simulink model "Simulink_Serial_Example"  (R2018b)
settings: Solver=VariableStepAuto  StartTime=0.0  StopTime=inf  RelTol=1e-3
undefined symbols (not defined in the file or in its folder): serial
libraries: instrumentlib x3
settings Model: Creator=root  LastModifiedBy=root

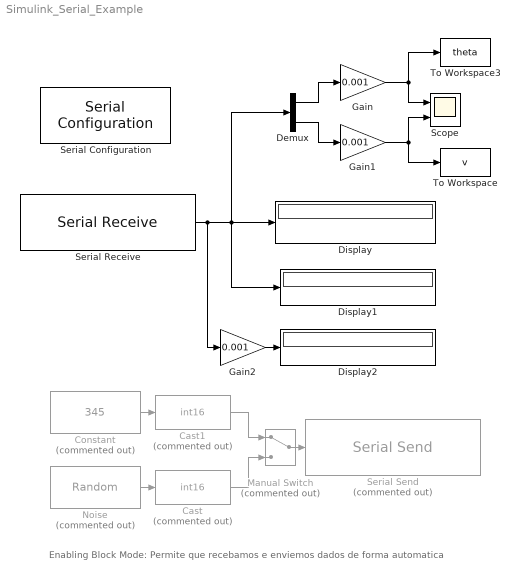
== system Simulink_Serial_Example ==
  note: Enabling Block Mode: Permite que recebamos e enviemos dados de forma automatica
  Cast : DataTypeConversion  Commented=on  OutDataTypeStr=int16
  Cast1 : DataTypeConversion  Commented=on  OutDataTypeStr=int16
  Constant : Constant  Commented=on  Value=345  VectorParams1D=off  OutDataTypeStr=int16  SampleTime=0.01
  Demux : Demux  Outputs=2
  Display : Display
      settings: Format=binary (Stored Integer)
  Display1 : Display
      settings: Format=decimal (Stored Integer)
  Display2 : Display
      settings: Format=decimal (Stored Integer)
  Gain : Gain  Gain=0.001
  Gain1 : Gain  Gain=0.001
  Gain2 : Gain  Gain=0.001
  Manual Switch : ManualSwitch  Commented=on
  Noise : UniformRandomNumber  Commented=on  Minimum=-32000  Maximum=32000  SampleTime=0.01
  Scope : Scope  NumInputPorts=2
  Serial Configuration : instrumentlib/Serial Configuration  Priority=-200000  ComPortMenu=/dev/ttyACM0  ComPort=/dev/ttyACM0  ObjConstructor=serial('/dev/ttyACM0');  BaudRate=115200  DataBits=8  Parity=none  StopBits=1  FlowControl=none  Timeout=10  ByteOrder=LittleEndian
  Serial Receive : instrumentlib/Serial Receive  ComPortMenu=/dev/ttyACM0  ComPort=/dev/ttyACM0  ObjConstructor=serial('/dev/ttyACM0');  Terminator=<none>  DataSize=2  DataType=int16  EnableBlockingMode=on  ActionDataUnavailable=Output last received value  CustomValue=0  SampleTime=0.025
  Serial Send : instrumentlib/Serial Send  Commented=on  ComPortMenu=<Please select a port...>  ComPort=/dev/cu.usbmodem14101  ObjConstructor=serial('/dev/cu.usbmodem14101');  Terminator=<none>  EnableBlockingMode=on
  To Workspace : ToWorkspace  VariableName=v  SaveFormat=Timeseries  SampleTime=-1
      settings: Save2DSignal=2-D array (concatenate along first dimension)
  To Workspace3 : ToWorkspace  VariableName=theta  SaveFormat=Timeseries  SampleTime=-1
      settings: Save2DSignal=2-D array (concatenate along first dimension)
  wires:
  Serial Receive/1 -> Gain2/1, Demux/1, Display1/1, Display/1
  Demux/1 -> Gain/1
  Gain/1 -> Scope/1, To Workspace3/1
  Demux/2 -> Gain1/1
  Gain1/1 -> To Workspace/1, Scope/2
  Manual Switch/1 -> Serial Send/1
  Noise/1 -> Cast/1
  Cast/1 -> Manual Switch/2
  Constant/1 -> Cast1/1
  Cast1/1 -> Manual Switch/1
  Gain2/1 -> Display2/1
